simulink model "turtlebot_waypoint2"  (R2017b)
settings: Solver=FixedStepDiscrete  StartTime=0.0  StopTime=inf  FixedStep=0.05  RelTol=1e-3  EnableMultiTasking=on
undefined symbols (not defined in the file): Angular, Linear
libraries: robotlib x3, simulink x1
settings Model: Creator=The MathWorks, Inc.  LastModifiedBy=jfmalia
settings DataIOCC: LimitDataPoints=on  SaveFormat=Array
settings OptimizationCC: DefaultUnderspecifiedDataType=single  LifeSpan=1  MaxStackSize=64
settings DebuggingCC: SolverPrmCheckMsg=warning  SFUnexpectedBacktrackingDiag=warning  SFNoUnconditionalDefaultTransitionDiag=warning  SFExecutionAtInitializationDiag=none
settings HardwareCC: ProdBitPerPointer=32  ProdBitPerSizeT=32  ProdBitPerPtrDiffT=32  ProdLargestAtomicFloat=None  ProdIntDivRoundTo=Undefined  ProdEndianess=Unspecified  ProdWordSize=32  ProdHWDeviceType=Generic->Unspecified (assume 32-bit Generic)  TargetHWDeviceType=Generic->Unspecified (assume 32-bit Generic)  UseEmbeddedCoderFeatures=off
settings ModelReferenceCC: PropagateSignalLabelsOutOfModel=off
settings RTWCC: SystemTargetFile=ert.tlc  HardwareBoard=Robot Operating System (ROS)  TLCOptions=-aInlineSetEventsForThisBaseRateFcn=TLC_FALSE -aSuppressMultiTaskScheduler=TLC_FALSE -aRateBasedStepFcn=0  TemplateMakefile=ert_default_tmf  Toolchain=Catkin  TargetLang=C++
settings CodeAppCC: StateflowObjectComments=on
settings ERTTargetCC: MultiwordLength=2048  ERTCustomFileBanners=off  MultiInstanceERTCode=on  CodeInterfacePackaging=C++ class  SupportContinuousTime=on  SupportNonInlinedSFcns=on  RemoveResetFunc=off  SupportVariableSizeSignals=on  ModelStepFunctionPrototypeControlCompliant=off  RootIOFormat=Structure reference  ConvertIfToSwitch=off  SuppressUnreachableDefaultCases=off
settings ConfigComp: CovMetricSettings=dw  CovHtmlReporting=on  CovSaveCumulativeToWorkspaceVar=on  CovSaveSingleToWorkspaceVar=on  CovExternalEMLEnable=off  CovSFcnEnable=off

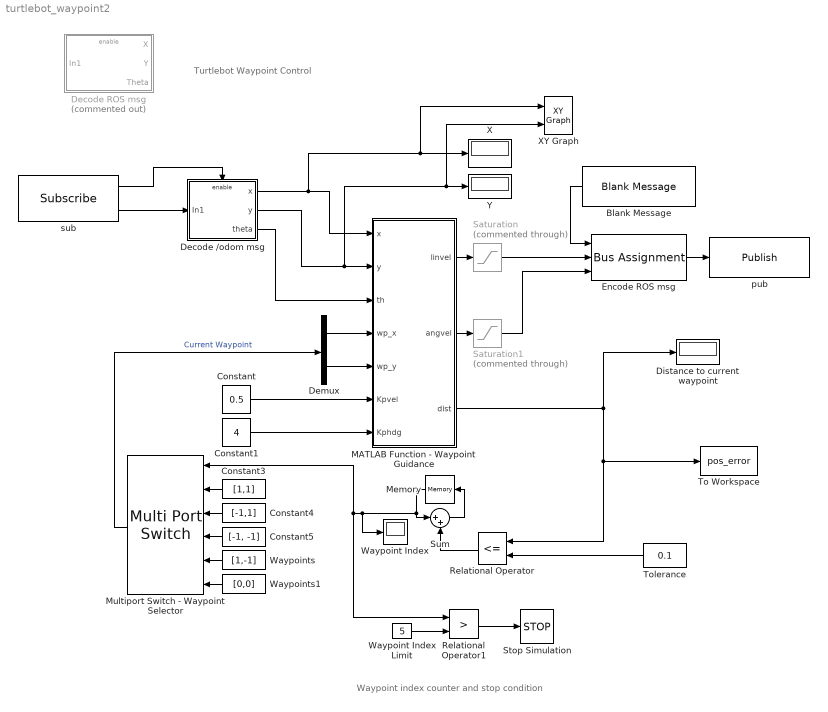
== system turtlebot_waypoint2 ==
  note: Waypoint index counter and stop condition
  note: Turtlebot Waypoint Control
  Blank Message : robotlib/Blank Message  SourceLibraryInfo=This block requires Robotics System Toolbox  messageType=geometry_msgs/Twist  SampleTime=inf
      settings: SourceProductBaseCode=RO
  Constant : Constant  Value=0.5
  Constant1 : Constant  Value=4
  Constant3 : Constant  Value=[1,1]
  Constant4 : Constant  Value=[-1,1]
  Constant5 : Constant  Value=[-1, -1]
  Decode /odom msg : Subsystem
  Decode ROS msg : Subsystem  Commented=on
  Demux : Demux  Outputs=2
  Distance to current waypoint : Display
  Encode ROS msg : BusAssignment  AssignedSignals=Linear.X,Angular.Z
  MATLAB Function - Waypoint Guidance : MATLAB Function  TreatAsAtomicUnit=on
  Memory : Memory  InitialCondition=1
  Multiport Switch - Waypoint Selector : MultiPortSwitch  Inputs=5  DiagnosticForDefault=Warning
  Relational Operator : RelationalOperator  Operator=<=  OutDataTypeStr=boolean  RndMeth=Simplest
  Relational Operator1 : RelationalOperator  Operator=>  OutDataTypeStr=boolean  RndMeth=Simplest
  Saturation : Saturate  Commented=through
  Saturation1 : Saturate  Commented=through  UpperLimit=1
  Stop Simulation : Stop
  Sum : Sum  Inputs=|++
  To Workspace : ToWorkspace  VariableName=pos_error  SaveFormat=Timeseries  SampleTime=-1
      settings: Decimation=2
  Tolerance : Constant  Value=0.1
  Waypoint Index : Display
  Waypoint Index Limit : Constant  Value=5
  Waypoints : Constant  Value=[1,-1]
  Waypoints1 : Constant  Value=[0,0]
  X : Display
  XY Graph : simulink/Sinks/XY Graph  xmin=-5  xmax=5  ymin=-5  ymax=5  st=-1
  Y : Display
  pub : robotlib/Publish  SourceLibraryInfo=This block requires Robotics System Toolbox  topicSource=Specify your own  topic=/cmd_vel  messageType=geometry_msgs/Twist  messageQueueLength=105
      settings: SourceProductBaseCode=RO
  "sub " : robotlib/Subscribe  SourceLibraryInfo=This block requires Robotics System Toolbox  topicSource=Specify your own  topic=/odom  messageType=nav_msgs/Odometry  sampleTime=-1  messageQueueLength=51
      settings: SourceProductBaseCode=RO
  wires:
  Encode ROS msg/1 -> pub/1
  Blank Message/1 -> Encode ROS msg/1
  MATLAB Function - Waypoint Guidance/1(linvel) -> Saturation/1
  MATLAB Function - Waypoint Guidance/2(angvel) -> Saturation1/1
  MATLAB Function - Waypoint Guidance/3(dist) -> Distance to current waypoint/1, To Workspace/1, Relational Operator/1
  Tolerance/1 -> Relational Operator/2
  Sum/1 -> Memory/1
  Memory/1 -> Waypoint Index/1, Relational Operator1/1, Multiport Switch - Waypoint Selector/1, Sum/1
  Constant3/1 -> Multiport Switch - Waypoint Selector/2
  Demux/1 -> MATLAB Function - Waypoint Guidance/4(wp_x)
  Demux/2 -> MATLAB Function - Waypoint Guidance/5(wp_y)
  Multiport Switch - Waypoint Selector/1 -> Demux/1  "Current Waypoint"
  Constant4/1 -> Multiport Switch - Waypoint Selector/3
  Constant5/1 -> Multiport Switch - Waypoint Selector/4
  Waypoints/1 -> Multiport Switch - Waypoint Selector/5
  Relational Operator/1 -> Sum/2
  Waypoint Index Limit/1 -> Relational Operator1/2
  Relational Operator1/1 -> Stop Simulation/1
  Waypoints1/1 -> Multiport Switch - Waypoint Selector/6
  Constant/1 -> MATLAB Function - Waypoint Guidance/6(Kpvel)
  Constant1/1 -> MATLAB Function - Waypoint Guidance/7(Kphdg)
  Decode /odom msg/2(y) -> XY Graph/2, Y/1, MATLAB Function - Waypoint Guidance/2(y)
  Decode /odom msg/1(x) -> XY Graph/1, X/1, MATLAB Function - Waypoint Guidance/1(x)
  Decode /odom msg/3("theta ") -> MATLAB Function - Waypoint Guidance/3(th)
  "sub "/2 -> Decode /odom msg/1(In1)
  "sub "/1 -> Decode /odom msg/Enable
  Saturation/1 -> Encode ROS msg/2
  Saturation1/1 -> Encode ROS msg/3

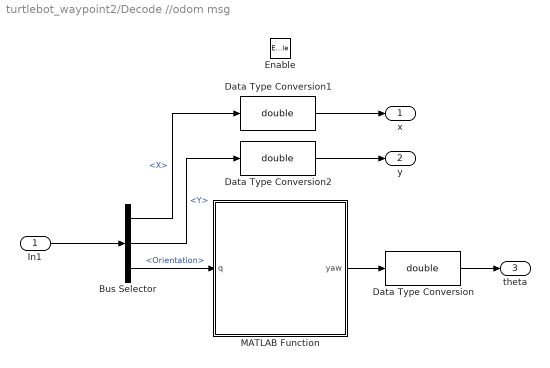
== system turtlebot_waypoint2/Decode //odom msg ==
  In1 : Inport
  Enable : EnablePort
  Bus Selector : BusSelector  OutputSignals=Pose.Pose.Position.X,Pose.Pose.Position.Y,Pose.Pose.Orientation
  Data Type Conversion : DataTypeConversion  OutDataTypeStr=double
  Data Type Conversion1 : DataTypeConversion  OutDataTypeStr=double
  Data Type Conversion2 : DataTypeConversion  OutDataTypeStr=double
  MATLAB Function : MATLAB Function  TreatAsAtomicUnit=on
  x : Outport
  y : Outport  Port=2
  "theta " : Outport  Port=3
  wires:
  Bus Selector/1 -> Data Type Conversion1/1  "<X>"
  MATLAB Function/1(yaw) -> Data Type Conversion/1
  Bus Selector/2 -> Data Type Conversion2/1  "<Y>"
  In1/1 -> Bus Selector/1
  Bus Selector/3 -> MATLAB Function/1(q)  "<Orientation>"
  Data Type Conversion2/1 -> y/1
  Data Type Conversion1/1 -> x/1
  Data Type Conversion/1 -> "theta "/1

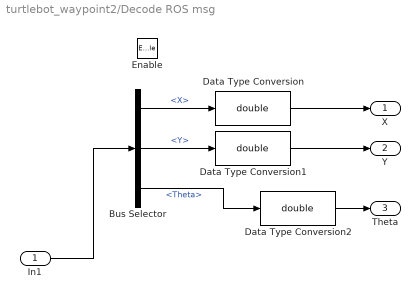
== system turtlebot_waypoint2/Decode ROS msg ==
  In1 : Inport
  Enable : EnablePort
  Bus Selector : BusSelector  DialogController=Simulink.DDGSource_BusSelector  OutputSignals=X,Y,Theta
  Data Type Conversion : DataTypeConversion  OutDataTypeStr=double
  Data Type Conversion1 : DataTypeConversion  OutDataTypeStr=double
  Data Type Conversion2 : DataTypeConversion  OutDataTypeStr=double
  X : Outport
  Y : Outport  Port=2
  Theta : Outport  Port=3
  wires:
  In1/1 -> Bus Selector/1
  Bus Selector/2 -> Data Type Conversion1/1  "<Y>"
  Bus Selector/1 -> Data Type Conversion/1  "<X>"
  Bus Selector/3 -> Data Type Conversion2/1  "<Theta>"
  Data Type Conversion/1 -> X/1
  Data Type Conversion1/1 -> Y/1
  Data Type Conversion2/1 -> Theta/1

== matlab function turtlebot_waypoint2/Decode //odom msg/MATLAB Function ==
  data: q input; yaw output
function yaw  = decode_odom_msg(q)
% q = Orientation.Pose.Pose;
angles = quat2eul([q.W q.X q.Y q.Z]);
yaw = angles(1);

== matlab function turtlebot_waypoint2/MATLAB Function - Waypoint Guidance ==
  data: linvel output; angvel output; x input; dist output; y input; th input; wp_x input; wp_y input; Kpvel input; Kphdg input
function [linvel,angvel,dist] = wpt_fcn(x,y,th,wp_x,wp_y,Kpvel,Kphdg)
% Function to implement waypoint guidance
% Inputs:
%  - x: Current X position
%  - y: Current Y position
%  - th: Current theta position
%  - wp_x: Current waypoint goals, X
%  - wp_y: Current waypoint goals, X
% Outputs:
%  - dist: Distance from current position to current waypoint goal
%  - angvel: Desired angular velocity [rad/s, clockwise]
%  - linvel: Desired linear velocity


% Distance from waypoint to current location
dist = sqrt((x-wp_x)^2+(y-wp_y)^2);

% Angle from current location to waypoint
course = atan2(wp_y-y,wp_x-x);

% Difference (error) between current turtle angle and desired angle
dhdg = course-th;

% Unwrap angle
while dhdg < -pi
    dhdg = dhdg + 2*pi;
end
while dhdg > pi
    dhdg = dhdg - 2*pi;
end

% Proportional Control 
% Gains
% Kpvel = 0.5;  % Proportional gain for velocity
% Kphdg = 2.0;  % Proportional gain for heading

% Specify commands to turtle
angvel=Kphdg*dhdg;
linvel = Kpvel*dist;

end
